simulink model "lab5_3"  (R2014b)
settings: Solver=ode45  StartTime=0.0  StopTime=100  RelTol=1e-3
values from neighbouring files (symbols this model uses):
  K = 0.6 * Kkr * (1 - (Tp/Tosc))    (= 5.7)    [lab5_1.m]
  Kz = 0.6 * Kkrz * (1 - (Tp/Toscz))    (= 2.67996)    [lab5_1.m]
  Mol = 0.1    [lab5_1.m]
  Mom = [1 -0.9]    [lab5_1.m]
  Ozl = 0.1    [lab5_1.m]
  Ozm = [1 -0.9 0 0 0]    [lab5_1.m]
  Td = 0.125 * ((Tosc/Tp)^2/((Tosc/Tp) - 1))    (= 0.5)    [lab5_1.m]
  Tdz = 0.125 * ((Toscz/Tp)^2/((Toscz/Tp) - 1))    (= 1.69836956522)    [lab5_1.m]
  Ti = 0.5 * ((Tosc/Tp) - 1)    (= 0.5)    [lab5_1.m]
  Tiz = 0.5 * ((Toscz/Tp) - 1)    (= 5.75)    [lab5_1.m]
  Tp = 1    [lab5_1.m]
libraries: simulink x8
settings Model: Creator=StudentPA  LastModifiedBy=StudentPA

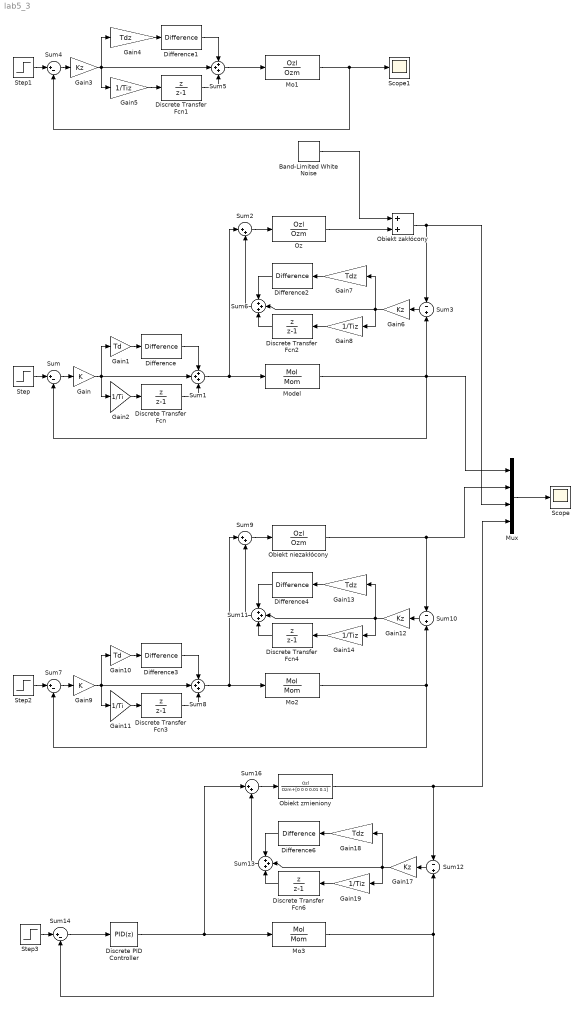
== system lab5_3 ==
  Band-Limited White Noise : simulink/Sources/Band-Limited White Noise  Cov=[0.01]  Ts=Tp  seed=[314159]
  Difference{,1..4,6} (6 alike) : simulink/Discrete/Difference  ICPrevInput=0.0  InputProcessing=Inherited  OutMin=[]  OutMax=[]  OutDataType=fixdt(1, 16)  OutScaling=2^-10  DoSatur=off
  Discrete Transfer Fcn{,2..4,6} (5 alike) : DiscreteTransferFcn  Numerator=[1 0]  Denominator=[1 -1]  SampleTime=Tp
  Discrete Transfer Fcn1 : DiscreteTransferFcn  Numerator=[1 0]  Denominator=[1 -1]
  Discrete PID Controller : simulink/Continuous/PID Controller  Controller=PID  TimeDomain=Discrete-time  SampleTime=1  IntegratorMethod=Forward Euler  FilterMethod=Forward Euler  Form=Parallel  P=1  I=1  D=0  N=100  InitialConditionSource=internal  InitialConditionForIntegrator=0  InitialConditionForFilter=0  ExternalReset=none  LimitOutput=off  UpperSaturationLimit=inf  LowerSaturationLimit=-inf  LinearizeAsGain=off  AntiWindupMode=none  Kb=1  TrackingMode=off  Kt=1  PParamMin=[]  PParamMax=[]  IParamMin=[]  IParamMax=[]  DParamMin=[]  DParamMax=[]  NParamMin=[]  NParamMax=[]  KbParamMin=[]  KbParamMax=[]  KtParamMin=[]  KtParamMax=[]  POutMin=[]  POutMax=[]  IOutMin=[]  IOutMax=[]  DOutMin=[]  DOutMax=[]  NOutMin=[]  NOutMax=[]  KbOutMin=[]  KbOutMax=[]  KtOutMin=[]  KtOutMax=[]  IntegratorOutMin=[]  IntegratorOutMax=[]  FilterOutMin=[]  FilterOutMax=[]  SumOutMin=[]  SumOutMax=[]  SumI1OutMin=[]  SumI1OutMax=[]  SumI2OutMin=[]  SumI2OutMax=[]  SumI3OutMin=[]  SumI3OutMax=[]  SumDOutMin=[]  SumDOutMax=[]  SaturationOutMin=[]  SaturationOutMax=[]  IntegratorContinuousStateAttributes=''  IntegratorStateMustResolveToSignalObject=off  IntegratorRTWStateStorageClass=Auto  FilterContinuousStateAttributes=''  FilterStateMustResolveToSignalObject=off  FilterRTWStateStorageClass=Auto  DifferentiatorICPrevScaledInput=0  DifferentiatorOutMin=[]  DifferentiatorOutMax=[]  UseFilter=on
  Gain : Gain  Gain=K  SampleTime=Tp
  Gain1 : Gain  Gain=Td
  Gain10 : Gain  Gain=Td
  Gain11 : Gain  Gain=1/Ti
  Gain12 : Gain  Gain=Kz
  Gain{4,7,13,18} (4 alike) : Gain  Gain=Tdz
  Gain{5,8,14,19} (4 alike) : Gain  Gain=1/Tiz
  Gain17 : Gain  Gain=Kz  SampleTime=Tp
  Gain2 : Gain  Gain=1/Ti
  Gain3 : Gain  Gain=Kz
  Gain6 : Gain  Gain=Kz
  Gain9 : Gain  Gain=K
  Mo1 : DiscreteTransferFcn  Numerator=Ozl  Denominator=Ozm
  Mo2 : DiscreteTransferFcn  Numerator=Mol  Denominator=Mom  SampleTime=Tp
  Mo3 : DiscreteTransferFcn  Numerator=Mol  Denominator=Mom  SampleTime=Tp
  Model : DiscreteTransferFcn  Numerator=Mol  Denominator=Mom  SampleTime=Tp
  Mux : Mux
  Obiekt niezakłócony : DiscreteTransferFcn  Numerator=Ozl  Denominator=Ozm  SampleTime=Tp
  Obiekt zakłócony : Sum
  Obiekt zmieniony : DiscreteTransferFcn  Numerator=Ozl  Denominator=Ozm+[0 0 0 0.01 0.1]  SampleTime=Tp
  Oz : DiscreteTransferFcn  Numerator=Ozl  Denominator=Ozm  SampleTime=Tp
  Scope : Scope
      settings: ShowLegends=on
  Scope1 : Scope
  Step{,1..3} (4 alike) : Step  Time=0  SampleTime=Tp
  Sum{,4,7,14} (4 alike) : Sum  Inputs=|+-
  Sum{1,5..6,8,11,13} (6 alike) : Sum  Inputs=+++
  Sum10 : Sum  Inputs=-|+
  Sum12 : Sum  Inputs=-|+
  Sum16 : Sum  Inputs=|++
  Sum2 : Sum  Inputs=|++
  Sum3 : Sum  Inputs=-|+
  Sum9 : Sum  Inputs=|++
  wires:
  Step/1 -> Sum/1
  Sum/1 -> Gain/1
  Sum1/1 -> Sum2/1, Model/1
  Gain1/1 -> Difference/1
  Gain/1 -> Sum1/2, Gain2/1, Gain1/1
  Gain2/1 -> Discrete Transfer Fcn/1
  Discrete Transfer Fcn/1 -> Sum1/3
  Difference/1 -> Sum1/1
  Mux/1 -> Scope/1
  Sum2/1 -> Oz/1
  Step1/1 -> Sum4/1
  Mo1/1 -> Scope1/1, Sum4/2
  Sum4/1 -> Gain3/1
  Sum5/1 -> Mo1/1
  Gain4/1 -> Difference1/1
  Gain3/1 -> Sum5/2, Gain4/1, Gain5/1
  Gain5/1 -> Discrete Transfer Fcn1/1
  Discrete Transfer Fcn1/1 -> Sum5/3
  Difference1/1 -> Sum5/1
  Gain7/1 -> Difference2/1
  Gain8/1 -> Discrete Transfer Fcn2/1
  Difference2/1 -> Sum6/1
  Discrete Transfer Fcn2/1 -> Sum6/3
  Gain6/1 -> Gain7/1, Gain8/1, Sum6/2
  Sum6/1 -> Sum2/2
  Sum3/1 -> Gain6/1
  Obiekt zakłócony/1 -> Mux/3, Sum3/1
  Oz/1 -> Obiekt zakłócony/2
  Band-Limited White Noise/1 -> Obiekt zakłócony/1
  Step2/1 -> Sum7/1
  Mo2/1 -> Sum10/2, Sum7/2
  Sum7/1 -> Gain9/1
  Sum8/1 -> Mo2/1, Sum9/1
  Gain10/1 -> Difference3/1
  Gain9/1 -> Gain10/1, Gain11/1, Sum8/2
  Gain11/1 -> Discrete Transfer Fcn3/1
  Discrete Transfer Fcn3/1 -> Sum8/3
  Difference3/1 -> Sum8/1
  Sum9/1 -> Obiekt niezakłócony/1
  Gain13/1 -> Difference4/1
  Gain14/1 -> Discrete Transfer Fcn4/1
  Difference4/1 -> Sum11/1
  Discrete Transfer Fcn4/1 -> Sum11/3
  Gain12/1 -> Sum11/2, Gain14/1, Gain13/1
  Sum11/1 -> Sum9/2
  Sum10/1 -> Gain12/1
  Obiekt niezakłócony/1 -> Mux/2, Sum10/1
  Step3/1 -> Sum14/1
  Mo3/1 -> Sum14/2, Sum12/2
  Sum14/1 -> Discrete PID Controller/1
  Sum16/1 -> Obiekt zmieniony/1
  Gain18/1 -> Difference6/1
  Gain19/1 -> Discrete Transfer Fcn6/1
  Difference6/1 -> Sum13/1
  Discrete Transfer Fcn6/1 -> Sum13/3
  Gain17/1 -> Gain18/1, Gain19/1, Sum13/2
  Sum13/1 -> Sum16/2
  Sum12/1 -> Gain17/1
  Obiekt zmieniony/1 -> Mux/4, Sum12/1
  Model/1 -> Sum/2, Mux/1, Sum3/2
  Discrete PID Controller/1 -> Sum16/1, Mo3/1
